simulink model "chap5_4sim"  (Simulink 3.00)
settings: Solver=ode45  StartTime=0.0  StopTime=1.5  RelTol=1e-3
settings Model: LastModifiedBy=liu

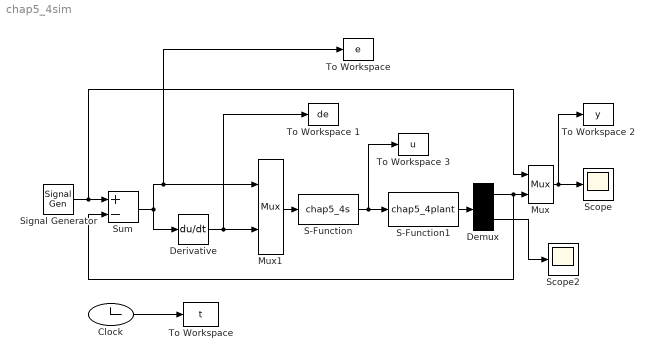
== system chap5_4sim ==
  Clock : Clock
  Demux : Demux  Outputs=2
  Derivative : Derivative
  Mux : Mux  Inputs=2
      settings: DisplayOption=none
  Mux1 : Mux  Inputs=2
      settings: DisplayOption=none
  S-Function : S-Function  FunctionName=chap5_4s  PortCounts=[]  SFunctionModules=''
  S-Function1 : S-Function  FunctionName=chap5_4plant  PortCounts=[]  SFunctionModules=''
  Scope : Scope
      settings: TimeRange=1  YMin=0.3  YMax=0.39  SaveToWorkspace=off  SaveName=ScopeData  MaxRows=500000
  Scope2 : Scope
      settings: TimeRange=1  YMin=-0.095  YMax=-0.015  SaveToWorkspace=off  SaveName=ScopeData  MaxRows=500000
  Signal Generator : SignalGenerator  WaveForm=sine  Amplitude=0.50  Frequency=3  Units=Hertz
  Sum : Sum  Inputs=+-  SaturateOnIntegerOverflow=on
  To Workspace : ToWorkspace  VariableName=t  SampleTime=-1  SaveFormat=Matrix
  "To Workspace " : ToWorkspace  VariableName=e  SampleTime=-1  SaveFormat=Matrix
  To Workspace 1 : ToWorkspace  VariableName=de  SampleTime=-1  SaveFormat=Matrix
  To Workspace 2 : ToWorkspace  VariableName=y  SampleTime=-1  SaveFormat=Matrix
  To Workspace 3 : ToWorkspace  VariableName=u  SampleTime=-1  SaveFormat=Matrix
  wires:
  Mux1/1 -> S-Function/1
  Derivative/1 -> Mux1/2, To Workspace 1/1
  S-Function/1 -> To Workspace 3/1, S-Function1/1
  Sum/1 -> Derivative/1, Mux1/1, "To Workspace "/1
  Signal Generator/1 -> Sum/1, Mux/1
  Demux/1 -> Mux/2, Sum/2
  Demux/2 -> Scope2/1
  Mux/1 -> Scope/1, To Workspace 2/1
  S-Function1/1 -> Demux/1
  Clock/1 -> To Workspace/1
